simulink model "junction_loop"  (R2020a)
settings: Solver=FixedStepDiscrete  StartTime=0.0  StopTime=0.1  FixedStep=0.1  RelTol=1e-3  EnableMultiTasking=on
settings Model: Creator=BEAR  LastModifiedBy=bzhan
settings SolverCC: AutoInsertRateTranBlk=on
settings DataIOCC: LimitDataPoints=on  ReturnWorkspaceOutputs=off
settings OptimizationCC: LifeSpan=inf
settings DebuggingCC: AllowSymbolicDim=off  SFUnexpectedBacktrackingDiag=warning  SFNoUnconditionalDefaultTransitionDiag=warning  SFExecutionAtInitializationDiag=none  ArithmeticOperatorsInVariantConditions=warning
settings SFSimCC: SimUseLocalCustomCode=off  CustomCodeUndefinedFunction=UseInterfaceOnly
settings RTWCC: RTWUseLocalCustomCode=off
settings CodeAppCC: StateflowObjectComments=on
settings GRTTargetCC: TargetLangStandard=C89/C90 (ANSI)
settings ConfigComp: CovMetricSettings=dw  CovHtmlReporting=on  CovSaveCumulativeToWorkspaceVar=on  CovSaveSingleToWorkspaceVar=on  CovShowResultsExplorer=off  CovExternalEMLEnable=off  CovSFcnEnable=off

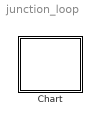
== system junction_loop ==
  Chart : Stateflow chart  TreatAsAtomicUnit=on

== stateflow chart junction_loop/Chart ==
  state A
  state B
  (junction 5) -> A [order 1] : [x==1]{t4}
  (default) -> A : {x=5}
  (junction 4) -> (junction 5) : {x=x-1;t1}
  A -> (junction 4)
  (junction 5) -> B [order 3] : {t3}
  (junction 5) -> (junction 4) [order 2] : [x>0]{t2}
  data: x local
  function t4:
    | function t4
    | 
    | fprintf("t4'")
  function t1:
    | function t1
    | 
    | fprintf("t1")
  function t2:
    | function t2
    | 
    | fprintf("t2")
  function t3:
    | function t3
    | 
    | fprintf("t3'")
